simulink model "VoltageSensorOffsetCalibrationComponent"  (R2025b)
settings: Solver=FixedStepDiscrete  StartTime=0.0  StopTime=10.0  RelTol=1e-3
settings Model: DataDictionary=TractionEmotorSoftwareArchInterfaceData.sldd  Creator=dakaihu  LastModifiedBy=dakaihu
settings OptimizationCC: ReuseModelBlockBuffer=off
settings RTWCC: GPUComputeCapability=3.5

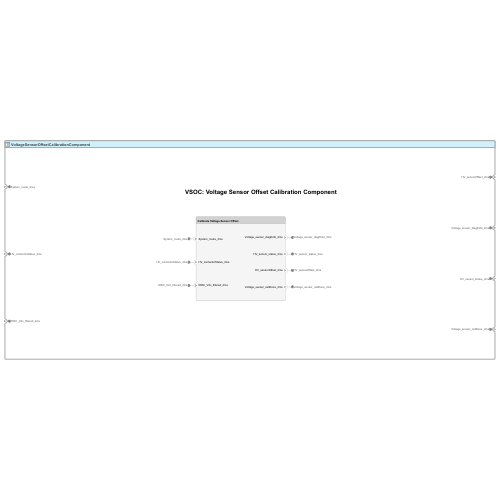
[thumbnail: Simulink's stored preview of the top-level diagram]
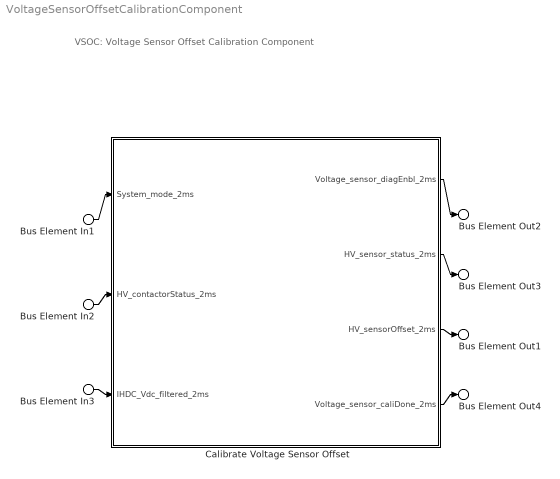
== system VoltageSensorOffsetCalibrationComponent ==
  note: VSOC: Voltage Sensor Offset Calibration Component
  Bus Element In1 : Inport  PortName=System_mode_2ms
  Bus Element In2 : Inport  Port=2  PortName=HV_contactorStatus_2ms
  Bus Element In3 : Inport  Port=3  PortName=IHDC_Vdc_filtered_2ms
  Calibrate Voltage Sensor Offset : Subsystem
      settings: PortSchema="{\"entries\":[{\"content\":{\"headerSize\":26,\"margin\":15,\"minimumSpacing\":25,\"sides\":[{\"content\":{\"connectorIds\":[\"In1\",\"In2\",\"In3\"]},\"type\":\"ConnectorPlacement.EquallySpacedRectSide\",\"uuid\":\"a0c63ab2-75fe-4bec-b2b0-6e2e00a1a5a4\"},{\"content\":{\"connectorIds\":[\"Out1\",\"Out2\",\"Out3\",\"Out4\"],\"side\":\"RIGHT\"},\"type\":\"ConnectorPlacement.EquallySpacedRectSide\",\"uuid\":\"05d605ea-8968-4533-a01c-bf4aae5caa93\"},{\"content\":{\"connectorIds\":[],\"side\":\"TOP\"},\"type\":\"ConnectorPlacement.EquallySpacedRectSide\",\"uuid\":\"27167c69-3967-4107-acce-f317c3d854af\"}]},\"type\":\"ConnectorPlacement.EquallySpacedConnector\",\"uuid\":\"c4d90da2-0f2a-4c00-bd24-85fead00d18f\"}],\"packageUris\":[\"http://schema.mathworks.com/mf0/Connector/R2020b\"],\"version\":\"1.0\"}"
  Bus Element Out1 : Outport  PortName=HV_sensorOffset_2ms
  Bus Element Out2 : Outport  Port=2  PortName=Voltage_sensor_diagEnbl_2ms
  Bus Element Out3 : Outport  Port=3  PortName=HV_sensor_status_2ms
  Bus Element Out4 : Outport  Port=4  PortName=Voltage_sensor_caliDone_2ms
  wires:
  Bus Element In1/1 -> Calibrate Voltage Sensor Offset/1(System_mode_2ms)
  Bus Element In2/1 -> Calibrate Voltage Sensor Offset/2(HV_contactorStatus_2ms)
  Bus Element In3/1 -> Calibrate Voltage Sensor Offset/3(IHDC_Vdc_filtered_2ms)
  Calibrate Voltage Sensor Offset/1(Voltage_sensor_diagEnbl_2ms) -> Bus Element Out2/1
  Calibrate Voltage Sensor Offset/2(HV_sensor_status_2ms) -> Bus Element Out3/1
  Calibrate Voltage Sensor Offset/3(HV_sensorOffset_2ms) -> Bus Element Out1/1
  Calibrate Voltage Sensor Offset/4(Voltage_sensor_caliDone_2ms) -> Bus Element Out4/1

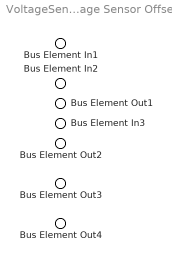
== system VoltageSensorOffsetCalibrationComponent/Calibrate Voltage Sensor Offset ==
  Bus Element In1 : Inport  PortName=System_mode_2ms
  Bus Element In2 : Inport  Port=2  PortName=HV_contactorStatus_2ms
  Bus Element In3 : Inport  Port=3  PortName=IHDC_Vdc_filtered_2ms
  Bus Element Out1 : Outport  PortName=Voltage_sensor_diagEnbl_2ms
  Bus Element Out2 : Outport  Port=2  PortName=HV_sensor_status_2ms
  Bus Element Out3 : Outport  Port=3  PortName=HV_sensorOffset_2ms
  Bus Element Out4 : Outport  Port=4  PortName=Voltage_sensor_caliDone_2ms
